simulink model "Project_Simulink_U3"  (R2020a)
settings: Solver=VariableStepAuto  StartTime=0.0  StopTime=50  RelTol=1e-3
libraries: simulink x17
settings Model: Creator=Manan  LastModifiedBy=Manan
settings DataIOCC: LoadExternalInput=on

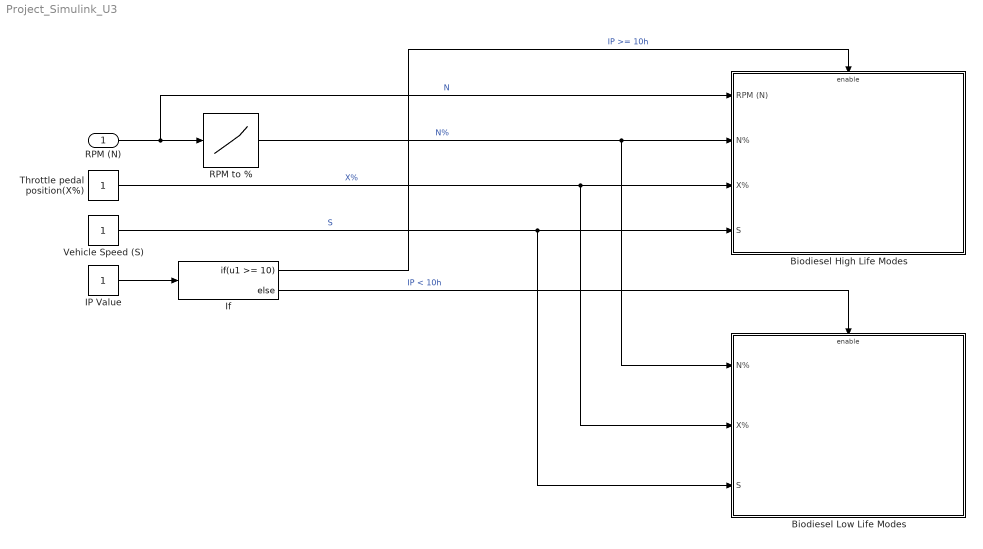
== system Project_Simulink_U3 ==
  RPM (N) : Inport
  Biodiesel High Life Modes : Subsystem  TreatAsAtomicUnit=on
  Biodiesel Low Life Modes : Subsystem  TreatAsAtomicUnit=on
  IP Value : Constant
  If : If  IfExpression=u1 >= 10
  RPM to % : Lookup_n-D  NumberOfTableDimensions=1  BreakpointsForDimension1=[800 6000]  Table=[0 100]  InternalRulePriority=Speed  RndMeth=Simplest  InputSameDT=on
  Throttle pedal position(X%) : Constant
  Vehicle Speed (S) : Constant
  wires:
  RPM (N)/1 -> RPM to %/1, Biodiesel High Life Modes/1(RPM (N))  "N"
  IP Value/1 -> If/1
  If/2 -> Biodiesel Low Life Modes/Enable  "IP < 10h"
  RPM to %/1 -> Biodiesel Low Life Modes/1(N%), Biodiesel High Life Modes/2(N%)  "N%"
  Throttle pedal position(X%)/1 -> Biodiesel Low Life Modes/2(X%), Biodiesel High Life Modes/3(X%)  "X%"
  Vehicle Speed (S)/1 -> Biodiesel Low Life Modes/3(S), Biodiesel High Life Modes/4(S)  "S"
  If/1 -> Biodiesel High Life Modes/Enable  "IP >= 10h"

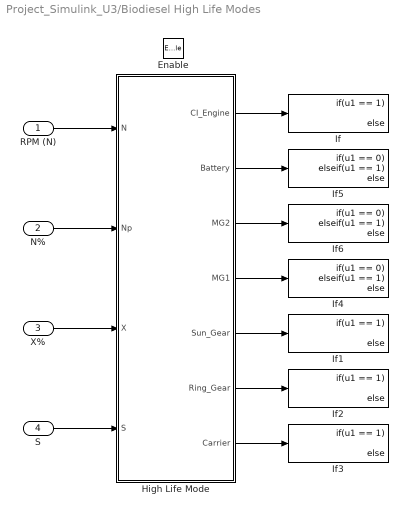
== system Project_Simulink_U3/Biodiesel High Life Modes ==
  RPM (N) : Inport
  N% : Inport  Port=2
  X% : Inport  Port=3
  S : Inport  Port=4
  Enable : EnablePort
  High Life Mode : Stateflow chart  TreatAsAtomicUnit=on
  If{,1..3} (4 alike) : If  IfExpression=u1 == 1
  If4 : If  IfExpression=u1 == 0  ElseIfExpressions=u1 == 1
  If5 : If  IfExpression=u1 == 0  ElseIfExpressions=u1 == 1
  If6 : If  IfExpression=u1 == 0  ElseIfExpressions=u1 == 1
  wires:
  S/1 -> High Life Mode/4(S)
  High Life Mode/6(Ring_Gear) -> If2/1
  High Life Mode/3(MG2) -> If6/1
  High Life Mode/1(CI_Engine) -> If/1
  High Life Mode/2(Battery) -> If5/1
  High Life Mode/4(MG1) -> If4/1
  High Life Mode/5(Sun_Gear) -> If1/1
  RPM (N)/1 -> High Life Mode/1(N)
  X%/1 -> High Life Mode/3(X)
  N%/1 -> High Life Mode/2(Np)
  High Life Mode/7(Carrier) -> If3/1

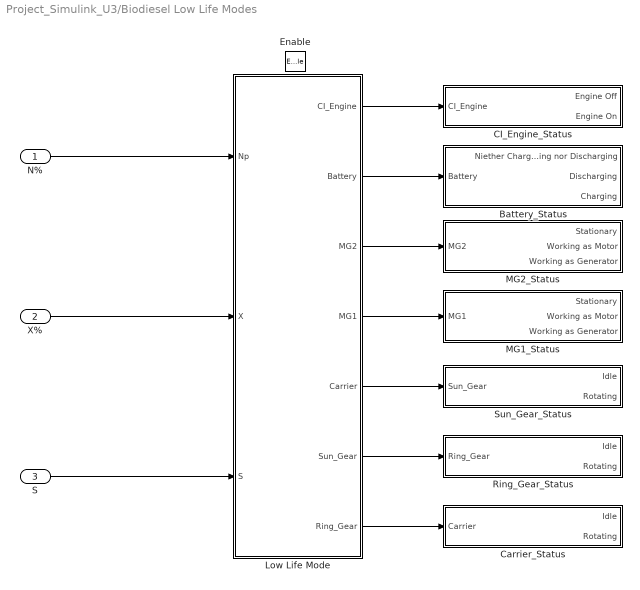
== system Project_Simulink_U3/Biodiesel Low Life Modes ==
  N% : Inport
  X% : Inport  Port=2
  S : Inport  Port=3
  Enable : EnablePort
  Battery_Status : Subsystem
  CI_Engine_Status : Subsystem
  Carrier_Status : Subsystem
  Low Life Mode : Stateflow chart  TreatAsAtomicUnit=on
  MG1_Status : Subsystem
  MG2_Status : Subsystem
  Ring_Gear_Status : Subsystem
  Sun_Gear_Status : Subsystem
  wires:
  S/1 -> Low Life Mode/3(S)
  N%/1 -> Low Life Mode/1(Np)
  X%/1 -> Low Life Mode/2(X)
  Low Life Mode/3(MG2) -> MG2_Status/1(MG2)
  Low Life Mode/2(Battery) -> Battery_Status/1(Battery)
  Low Life Mode/1(CI_Engine) -> CI_Engine_Status/1(CI_Engine)
  Low Life Mode/4(MG1) -> MG1_Status/1(MG1)
  Low Life Mode/5(Carrier) -> Sun_Gear_Status/1(Sun_Gear)
  Low Life Mode/6(Sun_Gear) -> Ring_Gear_Status/1(Ring_Gear)
  Low Life Mode/7(Ring_Gear) -> Carrier_Status/1(Carrier)

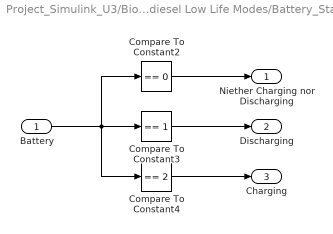
== system Project_Simulink_U3/Biodiesel Low Life Modes/Battery_Status ==
  Battery : Inport
  Compare To Constant2 : simulink/Logic and Bit Operations/Compare To Constant  relop===  const=0  OutDataTypeStr=boolean
  Compare To Constant3 : simulink/Logic and Bit Operations/Compare To Constant  relop===  const=1  OutDataTypeStr=boolean
  Compare To Constant4 : simulink/Logic and Bit Operations/Compare To Constant  relop===  const=2  OutDataTypeStr=boolean
  Niether Charging nor Discharging : Outport
  Discharging : Outport  Port=2
  Charging : Outport  Port=3
  wires:
  Compare To Constant2/1 -> Niether Charging nor Discharging/1
  Battery/1 -> Compare To Constant4/1, Compare To Constant2/1, Compare To Constant3/1
  Compare To Constant3/1 -> Discharging/1
  Compare To Constant4/1 -> Charging/1

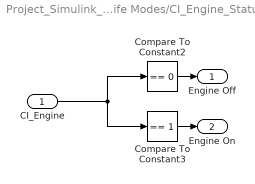
== system Project_Simulink_U3/Biodiesel Low Life Modes/CI_Engine_Status ==
  CI_Engine : Inport
  Compare To Constant2 : simulink/Logic and Bit Operations/Compare To Constant  relop===  const=0  OutDataTypeStr=boolean
  Compare To Constant3 : simulink/Logic and Bit Operations/Compare To Constant  relop===  const=1  OutDataTypeStr=boolean
  Engine Off : Outport
  Engine On : Outport  Port=2
  wires:
  Compare To Constant3/1 -> Engine On/1
  CI_Engine/1 -> Compare To Constant3/1, Compare To Constant2/1
  Compare To Constant2/1 -> Engine Off/1

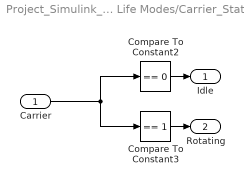
== system Project_Simulink_U3/Biodiesel Low Life Modes/Carrier_Status ==
  Carrier : Inport
  Compare To Constant2 : simulink/Logic and Bit Operations/Compare To Constant  relop===  const=0  OutDataTypeStr=boolean
  Compare To Constant3 : simulink/Logic and Bit Operations/Compare To Constant  relop===  const=1  OutDataTypeStr=boolean
  Idle : Outport
  Rotating : Outport  Port=2
  wires:
  Compare To Constant2/1 -> Idle/1
  Carrier/1 -> Compare To Constant2/1, Compare To Constant3/1
  Compare To Constant3/1 -> Rotating/1

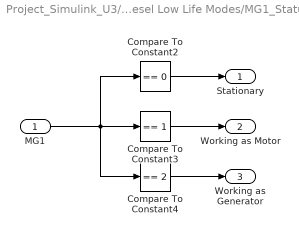
== system Project_Simulink_U3/Biodiesel Low Life Modes/MG1_Status ==
  MG1 : Inport
  Compare To Constant2 : simulink/Logic and Bit Operations/Compare To Constant  relop===  const=0  OutDataTypeStr=boolean
  Compare To Constant3 : simulink/Logic and Bit Operations/Compare To Constant  relop===  const=1  OutDataTypeStr=boolean
  Compare To Constant4 : simulink/Logic and Bit Operations/Compare To Constant  relop===  const=2  OutDataTypeStr=boolean
  Stationary : Outport
  Working as Motor : Outport  Port=2
  Working as Generator : Outport  Port=3
  wires:
  Compare To Constant2/1 -> Stationary/1
  MG1/1 -> Compare To Constant4/1, Compare To Constant2/1, Compare To Constant3/1
  Compare To Constant3/1 -> Working as Motor/1
  Compare To Constant4/1 -> Working as Generator/1

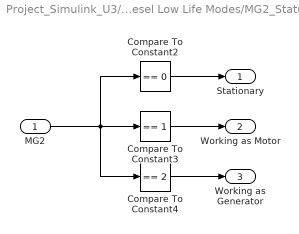
== system Project_Simulink_U3/Biodiesel Low Life Modes/MG2_Status ==
  MG2 : Inport
  Compare To Constant2 : simulink/Logic and Bit Operations/Compare To Constant  relop===  const=0  OutDataTypeStr=boolean
  Compare To Constant3 : simulink/Logic and Bit Operations/Compare To Constant  relop===  const=1  OutDataTypeStr=boolean
  Compare To Constant4 : simulink/Logic and Bit Operations/Compare To Constant  relop===  const=2  OutDataTypeStr=boolean
  Stationary : Outport
  Working as Motor : Outport  Port=2
  Working as Generator : Outport  Port=3
  wires:
  Compare To Constant4/1 -> Working as Generator/1
  Compare To Constant3/1 -> Working as Motor/1
  MG2/1 -> Compare To Constant3/1, Compare To Constant2/1, Compare To Constant4/1
  Compare To Constant2/1 -> Stationary/1

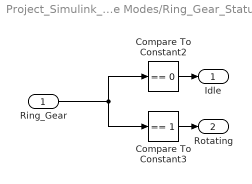
== system Project_Simulink_U3/Biodiesel Low Life Modes/Ring_Gear_Status ==
  Ring_Gear : Inport
  Compare To Constant2 : simulink/Logic and Bit Operations/Compare To Constant  relop===  const=0  OutDataTypeStr=boolean
  Compare To Constant3 : simulink/Logic and Bit Operations/Compare To Constant  relop===  const=1  OutDataTypeStr=boolean
  Idle : Outport
  Rotating : Outport  Port=2
  wires:
  Compare To Constant3/1 -> Rotating/1
  Ring_Gear/1 -> Compare To Constant3/1, Compare To Constant2/1
  Compare To Constant2/1 -> Idle/1

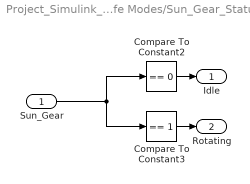
== system Project_Simulink_U3/Biodiesel Low Life Modes/Sun_Gear_Status ==
  Sun_Gear : Inport
  Compare To Constant2 : simulink/Logic and Bit Operations/Compare To Constant  relop===  const=0  OutDataTypeStr=boolean
  Compare To Constant3 : simulink/Logic and Bit Operations/Compare To Constant  relop===  const=1  OutDataTypeStr=boolean
  Idle : Outport
  Rotating : Outport  Port=2
  wires:
  Compare To Constant2/1 -> Idle/1
  Sun_Gear/1 -> Compare To Constant2/1, Compare To Constant3/1
  Compare To Constant3/1 -> Rotating/1

== stateflow chart Project_Simulink_U3/Biodiesel Low Life Modes/Low Life Mode ==
  state Existing_Mode
    entry:
  state LightLoad_Mode
    entry:
    CI_Engine = 1
    Battery = 0
    MG2 = 0
    MG1 = 0
    exit:
    Sun_Gear = 0
    Carrier = 1
    Ring_Gear = 1
  state Acceleration_Mode
    entry:
    CI_Engine = 1
    Battery = 1
    MG2 = 1
    MG1 = 2
    exit:
    Sun_Gear = 1
    Carrier = 1
    Ring_Gear = 1
  state Cruising_Mode
    entry:
    CI_Engine = 1
    Battery = 2
    MG2 = 0
    MG1 = 2
    exit:
    Sun_Gear = 1
    Carrier = 1
    Ring_Gear = 1
  state Braking_Mode
    entry:
    CI_Engine = 1
    Battery = 2
    MG2 = 2
    MG1 = 0
    exit:
    Sun_Gear = 0
    Carrier = 1
    Ring_Gear = 1
  state BatteryCharging_Mode_Standstill_Mode
    entry:
    CI_Engine = 1
    Battery = 2
    MG2 = 0
    MG1 = 2
    exit:
    Sun_Gear = 1
    Carrier = 1
    Ring_Gear = 0
  (default) -> Existing_Mode
  Existing_Mode -> LightLoad_Mode [order 1] : [Np == 0 && X >= 0 && X <= 35 ]
  Existing_Mode -> Acceleration_Mode [order 2] : [((Np+5) < X) && (35 < X <=100)]
  Existing_Mode -> Cruising_Mode [order 3] : [(Np-10) < X < (Np+10)]
  Existing_Mode -> Braking_Mode [order 4] : [S ~= 0 && X == 0]
  Existing_Mode -> BatteryCharging_Mode_Standstill_Mode [order 5] : [Np == 0 && S == 0 && X == 0 || S == 0]
  data: Np input; X input; S input; CI_Engine output; Battery output; MG2 output; MG1 output; Carrier output; Sun_Gear output; Ring_Gear output

== stateflow chart Project_Simulink_U3/Biodiesel High Life Modes/High Life Mode ==
  state Existing_Mode
    entry:
  state Standstill_Mode
    entry:
    CI_Engine = 0
    Battery = 0
    MG2 = 0
    MG1 = 0
  state LightLoad_Mode
    entry:
    CI_Engine = 0
    Battery = 1
    MG2 = 1
    MG1 = 0
    Sun_Gear = 1
    Carrier = 0
    Ring_Gear = 1
  state Acceleration_Mode
    entry:
    CI_Engine = 1
    Battery = 1
    MG2 = 1
    MG1 = 0
    Sun_Gear = 0
    Carrier = 1
    Ring_Gear = 1
  state Cruising_Mode
    entry:
    CI_Engine = 1
    Battery = 1
    MG2 = 1
    MG1 = 0
    Sun_Gear = 0
    Carrier = 1
    Ring_Gear = 1
  state Braking_Mode
    entry:
    CI_Engine = 1
    Battery = 2
    MG2 = 2
    MG1 = 0
    Sun_Gear = 1
    Carrier = 1
    Ring_Gear = 1
  state BatteryCharging_Mode
    entry:
    CI_Engine = 1
    Battery = 2
    MG2 = 0
    MG1 = 2
    Sun_Gear = 1
    Carrier = 1
    Ring_Gear = 0
  (default) -> Existing_Mode
  Existing_Mode -> Standstill_Mode [order 1] : [S == 0]
  Existing_Mode -> LightLoad_Mode [order 2] : [N == 0 && X >= 0 && X <= 35 ]
  Existing_Mode -> Acceleration_Mode [order 3] : [((Np+5) < X) && (35 < X <=100)]
  Existing_Mode -> Cruising_Mode [order 4] : [(Np-10) < X < (Np+10)]
  Existing_Mode -> Braking_Mode [order 5] : [S ~= 0 && X == 0]
  Existing_Mode -> BatteryCharging_Mode [order 6] : [Np == 0 && S == 0 && X == 0]
  data: N input; Np input; X input; S input; CI_Engine output; Battery output; MG2 output; MG1 output; Sun_Gear output; Ring_Gear output; Carrier output
